simulink model "observer_test"  (R2022a)
settings: Solver=VariableStepAuto  StartTime=0.0  StopTime=10.0  RelTol=1e-3
values from neighbouring files (symbols this model uses):
  A = ss_d.A    [LQR_sim.m]    (also in observer_design.m = A(1:2,1:2))
  Aobs = A-L*C    [observer_design.m]
  B = ss_d.B    [LQR_sim.m]    (also in observer_design.m = B(1:2,1))
  Bobs = [B L]    [observer_design.m]
  C = ss_d.C    [LQR_sim.m]    (also in observer_design.m = C(1,1:2))
  Cobs = eye(2)    [observer_design.m]
  Dobs = [0,0 ... (first row only)    [observer_design.m]
  K = -acker(A,B,poles)    [observer_design.m]
settings Model: Creator=michi  LastModifiedBy=michi

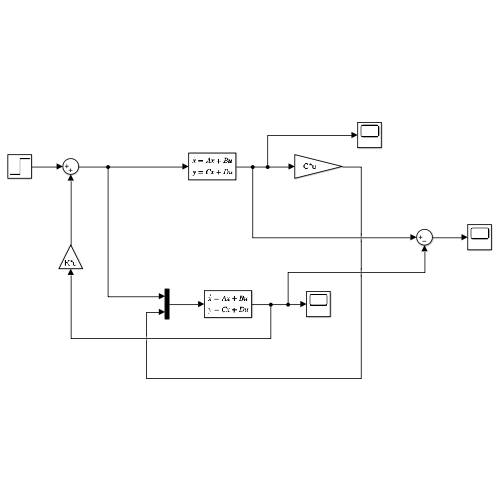
[thumbnail: Simulink's stored preview of the top-level diagram]
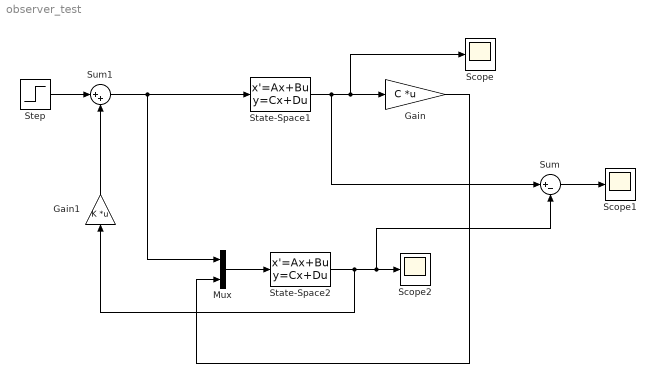
== system observer_test ==
  Gain : Gain  Gain=C  Multiplication=Matrix(K*u)
  Gain1 : Gain  Gain=K  Multiplication=Matrix(K*u)
  Mux : Mux  Inputs=2
  Scope : Scope
  Scope1 : Scope
  Scope2 : Scope
  State-Space1 : StateSpace  A=A  B=B  C=eye(2)  D=[0;0]  InitialCondition=[10 -10]'
  State-Space2 : StateSpace  A=Aobs  B=Bobs  C=Cobs  D=Dobs  InitialCondition=0
  Step : Step  SampleTime=0
  Sum : Sum  Inputs=|+-
  Sum1 : Sum  Inputs=|++
  wires:
  Mux/1 -> State-Space2/1
  State-Space1/1 -> Sum/1, Scope/1, Gain/1
  Step/1 -> Sum1/1
  Sum1/1 -> Mux/1, State-Space1/1
  State-Space2/1 -> Gain1/1, Sum/2, Scope2/1
  Gain1/1 -> Sum1/2
  Gain/1 -> Mux/2
  Sum/1 -> Scope1/1
